simulink model "fifth"  (R2018a)
settings: Solver=VariableStepAuto  StartTime=0.0  StopTime=10.0  RelTol=1e-3
values from neighbouring files (symbols this model uses):
  ki = 0.01    [matlab.mat]
  kp = 0.2    [matlab.mat]
  Qs = 0.125    [matlab.mat]
  R = 1.6    [matlab.mat]
settings Model: Creator=Master  LastModifiedBy=Master

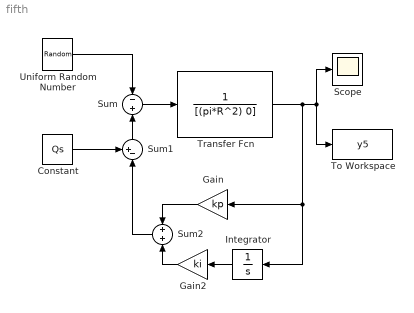
== system fifth ==
  Constant : Constant  Value=Qs
  Gain : Gain  Gain=kp
  Gain2 : Gain  Gain=ki
  Integrator : Integrator
  Scope : Scope
  Sum : Sum  Inputs=-|+
  Sum1 : Sum  Inputs=+-|
  Sum2 : Sum  Inputs=+|+
  To Workspace : ToWorkspace  VariableName=y5  SaveFormat=Timeseries  SampleTime=-1
  Transfer Fcn : TransferFcn  Denominator=[(pi*R^2) 0]
  Uniform Random Number : UniformRandomNumber  SampleTime=0.1
  wires:
  Uniform Random Number/1 -> Sum/1
  Constant/1 -> Sum1/1
  Sum/1 -> Transfer Fcn/1
  Transfer Fcn/1 -> Integrator/1, Gain/1, To Workspace/1, Scope/1
  Sum1/1 -> Sum/2
  Gain/1 -> Sum2/1
  Gain2/1 -> Sum2/2
  Integrator/1 -> Gain2/1
  Sum2/1 -> Sum1/2
